simulink model "EncTest"  (R2022b)
settings: Solver=FixedStepDiscrete  StartTime=0.0  StopTime=inf  FixedStep=0.001  RelTol=1e-3
settings Model: DataDictionary=MCU_Input_Sldd.sldd  Creator=ZYH  LastModifiedBy=ZYH
settings OptimizationCC: DefaultParameterBehavior=Inlined  DefaultUnderspecifiedDataType=single  EnhancedBackFolding=on  PassReuseOutputArgsAs=Individual arguments  ZeroExternalMemoryAtStartup=off  ZeroInternalMemoryAtStartup=off  OptimizeBlockOrder=speed  DifferentSizesBufferReuse=on  OptimizationCustomize=off  EfficientTunableParamExpr=on
settings DebuggingCC: ParameterTunabilityLossMsg=error
settings SFSimCC: MATLABDynamicMemAlloc=off
settings RTWCC: Description=Embedded Coder  SystemTargetFile=ert.tlc  GenCodeOnly=on  TemplateMakefile=ert_default_tmf
settings CodeAppCC: IgnoreCustomStorageClasses=off  MaxIdLength=40  OperatorAnnotations=on  SimulinkDataObjDesc=on  SFDataObjDesc=on  SimulinkBlockComments=off
settings ERTTargetCC: TargetLangStandard=C99 (ISO)  GenerateSampleERTMain=on  InlinedParameterPlacement=NonHierarchical  ERTCustomFileTemplate=example_file_process.tlc

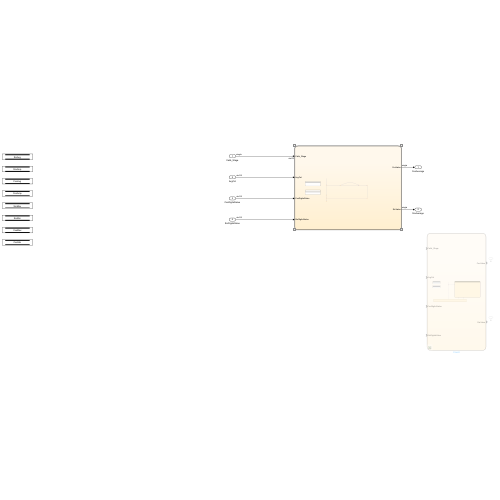
[thumbnail: Simulink's stored preview of the top-level diagram]
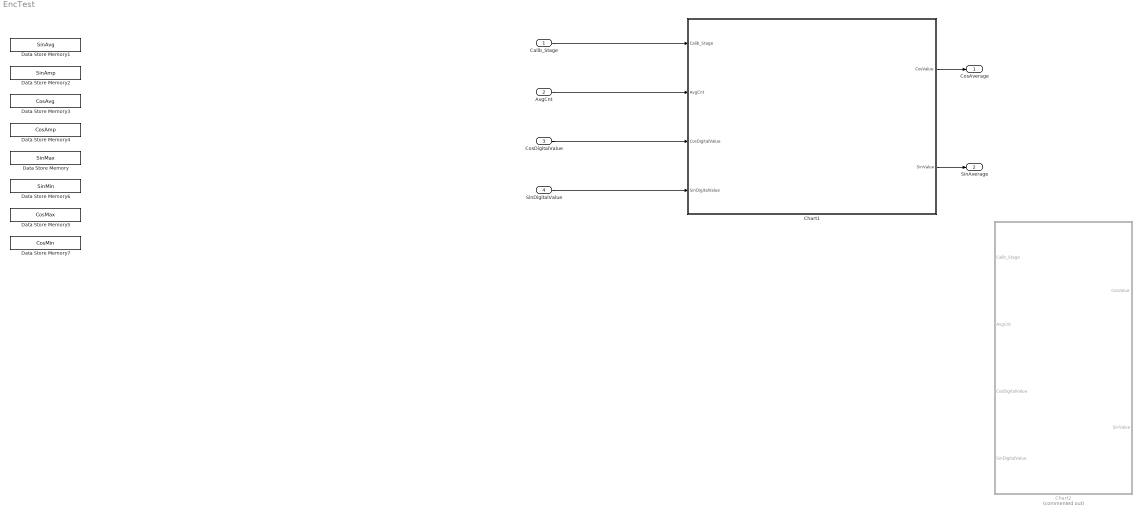
== system EncTest ==
  Calib_Stage : Inport
  AvgCnt : Inport  Port=2
  CosDigitalValue : Inport  Port=3
  SinDigitalValue : Inport  Port=4
  Chart1 : Stateflow chart  TreatAsAtomicUnit=on
      settings: RTWSystemCode=Nonreusable function
  Chart2 : Stateflow chart  Commented=on  TreatAsAtomicUnit=on
      settings: RTWSystemCode=Nonreusable function
  Data Store Memory : DataStoreMemory  DataStoreName=SinMax  WriteAfterWriteMsg=warning  InitialValue=2048  ShowAdditionalParam=off
  Data Store Memory1 : DataStoreMemory  DataStoreName=SinAvg  WriteAfterWriteMsg=warning  InitialValue=ParamCfg_Sinavg_u16  ShowAdditionalParam=off  OutDataTypeStr=uint16  StateMustResolveToSignalObject=on
  Data Store Memory2 : DataStoreMemory  DataStoreName=SinAmp  WriteAfterWriteMsg=warning  InitialValue=ParamCfg_Sinamp_u16  ShowAdditionalParam=off  OutDataTypeStr=uint16  StateMustResolveToSignalObject=on
  Data Store Memory3 : DataStoreMemory  DataStoreName=CosAvg  WriteAfterWriteMsg=warning  InitialValue=ParamCfg_Cosavg_u16  ShowAdditionalParam=off  OutDataTypeStr=uint16  StateMustResolveToSignalObject=on
  Data Store Memory4 : DataStoreMemory  DataStoreName=CosAmp  WriteAfterWriteMsg=warning  InitialValue=ParamCfg_Cosamp_u16  ShowAdditionalParam=off  OutDataTypeStr=uint16  StateMustResolveToSignalObject=on
  Data Store Memory5 : DataStoreMemory  DataStoreName=CosMax  WriteAfterWriteMsg=warning  InitialValue=2048  ShowAdditionalParam=off
  Data Store Memory6 : DataStoreMemory  DataStoreName=SinMin  WriteAfterWriteMsg=warning  InitialValue=2048  ShowAdditionalParam=off
  Data Store Memory7 : DataStoreMemory  DataStoreName=CosMin  WriteAfterWriteMsg=warning  InitialValue=2048  ShowAdditionalParam=off
  CosAverage : Outport
  SinAverage : Outport  Port=2
  wires:
  Chart1/1(CosValue) -> CosAverage/1
  Chart1/2(SinValue) -> SinAverage/1
  Calib_Stage/1 -> Chart1/1(Calib_Stage)
  AvgCnt/1 -> Chart1/2(AvgCnt)
  CosDigitalValue/1 -> Chart1/3(CosDigitalValue)
  SinDigitalValue/1 -> Chart1/4(SinDigitalValue)

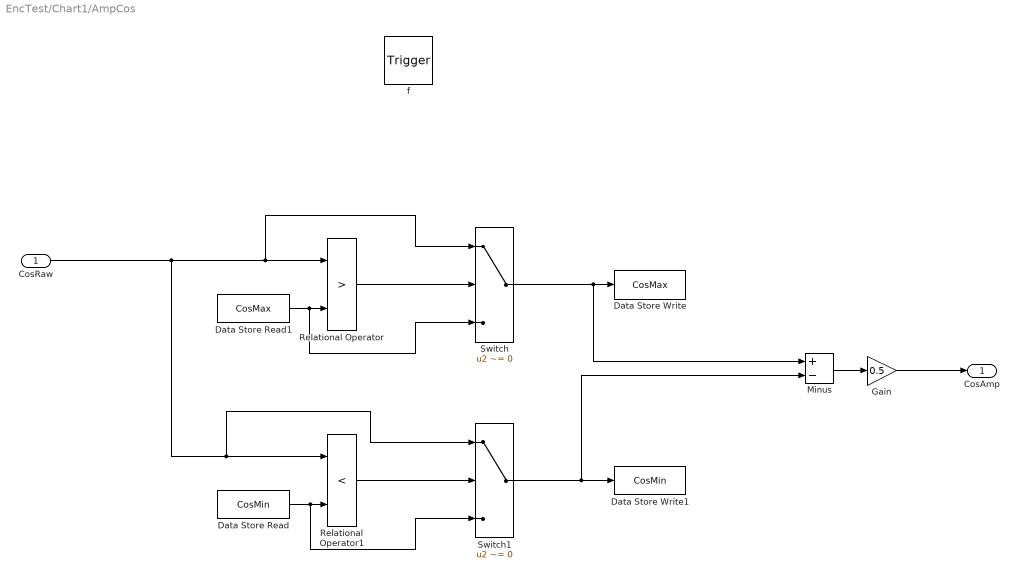
== system EncTest/Chart1/AmpCos ==
  CosRaw : Inport  OutDataTypeStr=uint16  PortDimensions=1
  f : TriggerPort  TriggerType=function-call  VariantControl=(inherit)
      settings: CopyFcn=Stateflow.SLINSF.SimulinkMan.removeBlockPreDeleteFcn  PreDeleteFcn=Stateflow.SLINSF.SimulinkMan.unsafePredeleteFcn
  Data Store Read : DataStoreRead  DataStoreName=CosMin  IndexOptions=Index vector (dialog)  Indices=1  OutputSizes=1
  Data Store Read1 : DataStoreRead  DataStoreName=CosMax  IndexOptions=Index vector (dialog)  Indices=1  OutputSizes=1
  Data Store Write : DataStoreWrite  DataStoreName=CosMax  IndexOptions=Index vector (dialog)  Indices=1  OutputSizes=1
  Data Store Write1 : DataStoreWrite  DataStoreName=CosMin  IndexOptions=Index vector (dialog)  Indices=1  OutputSizes=1
  Gain : Gain  Gain=0.5  ParamDataTypeStr=single  OutDataTypeStr=single
  Minus : Sum  Inputs=+-
  Relational Operator : RelationalOperator  Operator=>  OutDataTypeStr=boolean  RndMeth=Simplest  InputSameDT=off
  Relational Operator1 : RelationalOperator  Operator=<  OutDataTypeStr=boolean  RndMeth=Simplest  InputSameDT=off
  Switch : Switch  Criteria=u2 ~= 0  SaturateOnIntegerOverflow=off  InputSameDT=off
  Switch1 : Switch  Criteria=u2 ~= 0  SaturateOnIntegerOverflow=off  InputSameDT=off
  CosAmp : Outport  OutDataTypeStr=single
  wires:
  CosRaw/1 -> Switch1/1, Relational Operator1/1, Switch/1, Relational Operator/1
  Data Store Read1/1 -> Switch/3, Relational Operator/2
  Relational Operator/1 -> Switch/2
  Switch/1 -> Minus/1, Data Store Write/1
  Data Store Read/1 -> Switch1/3, Relational Operator1/2
  Relational Operator1/1 -> Switch1/2
  Switch1/1 -> Minus/2, Data Store Write1/1
  Minus/1 -> Gain/1
  Gain/1 -> CosAmp/1

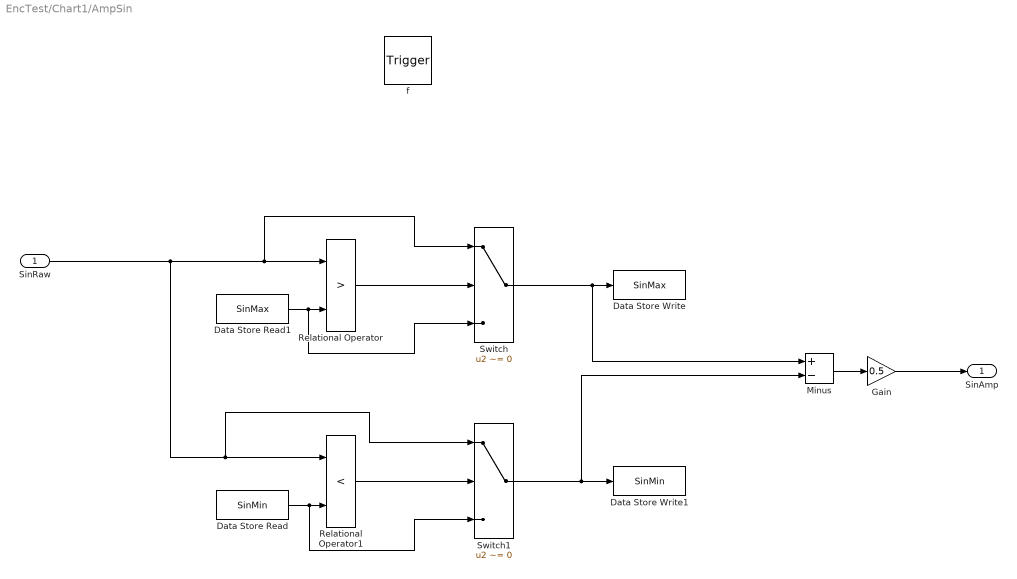
== system EncTest/Chart1/AmpSin ==
  SinRaw : Inport  OutDataTypeStr=uint16  PortDimensions=1
  f : TriggerPort  TriggerType=function-call  VariantControl=(inherit)
      settings: CopyFcn=Stateflow.SLINSF.SimulinkMan.removeBlockPreDeleteFcn  PreDeleteFcn=Stateflow.SLINSF.SimulinkMan.unsafePredeleteFcn
  Data Store Read : DataStoreRead  DataStoreName=SinMin  IndexOptions=Index vector (dialog)  Indices=1  OutputSizes=1
  Data Store Read1 : DataStoreRead  DataStoreName=SinMax  IndexOptions=Index vector (dialog)  Indices=1  OutputSizes=1
  Data Store Write : DataStoreWrite  DataStoreName=SinMax  IndexOptions=Index vector (dialog)  Indices=1  OutputSizes=1
  Data Store Write1 : DataStoreWrite  DataStoreName=SinMin  IndexOptions=Index vector (dialog)  Indices=1  OutputSizes=1
  Gain : Gain  Gain=0.5  ParamDataTypeStr=single  OutDataTypeStr=single
  Minus : Sum  Inputs=+-
  Relational Operator : RelationalOperator  Operator=>  OutDataTypeStr=boolean  RndMeth=Simplest  InputSameDT=off
  Relational Operator1 : RelationalOperator  Operator=<  OutDataTypeStr=boolean  RndMeth=Simplest  InputSameDT=off
  Switch : Switch  Criteria=u2 ~= 0  SaturateOnIntegerOverflow=off  InputSameDT=off
  Switch1 : Switch  Criteria=u2 ~= 0  SaturateOnIntegerOverflow=off  InputSameDT=off
  SinAmp : Outport  OutDataTypeStr=single  PortDimensions=1
  wires:
  SinRaw/1 -> Switch1/1, Relational Operator1/1, Switch/1, Relational Operator/1
  Data Store Read1/1 -> Switch/3, Relational Operator/2
  Relational Operator/1 -> Switch/2
  Switch/1 -> Minus/1, Data Store Write/1
  Data Store Read/1 -> Switch1/3, Relational Operator1/2
  Relational Operator1/1 -> Switch1/2
  Switch1/1 -> Minus/2, Data Store Write1/1
  Minus/1 -> Gain/1
  Gain/1 -> SinAmp/1

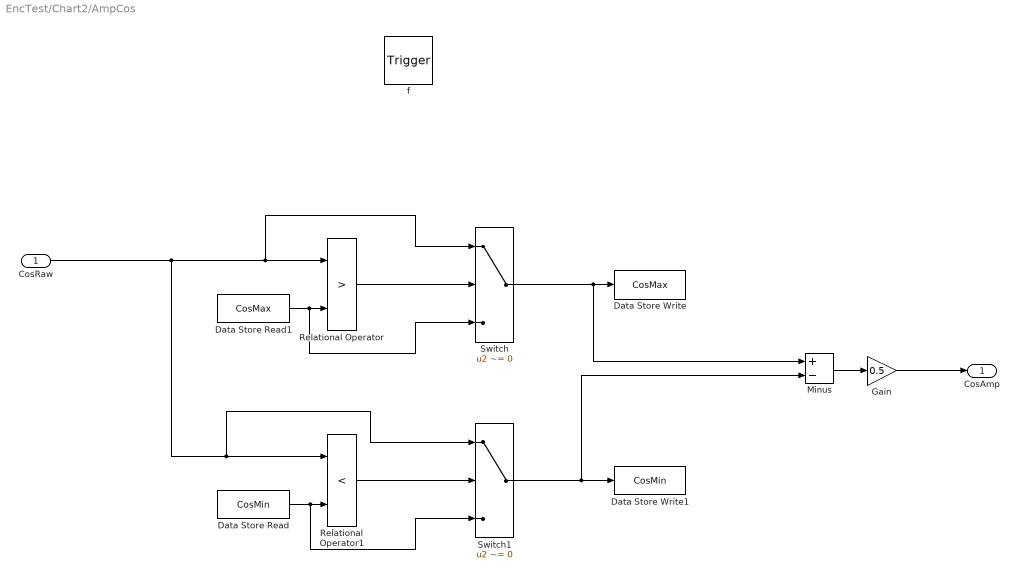
== system EncTest/Chart2/AmpCos ==
  CosRaw : Inport  OutDataTypeStr=uint16  PortDimensions=1
  f : TriggerPort  TriggerType=function-call  VariantControl=(inherit)
      settings: CopyFcn=Stateflow.SLINSF.SimulinkMan.removeBlockPreDeleteFcn  PreDeleteFcn=Stateflow.SLINSF.SimulinkMan.unsafePredeleteFcn
  Data Store Read : DataStoreRead  DataStoreName=CosMin  IndexOptions=Index vector (dialog)  Indices=1  OutputSizes=1
  Data Store Read1 : DataStoreRead  DataStoreName=CosMax  IndexOptions=Index vector (dialog)  Indices=1  OutputSizes=1
  Data Store Write : DataStoreWrite  DataStoreName=CosMax  IndexOptions=Index vector (dialog)  Indices=1  OutputSizes=1
  Data Store Write1 : DataStoreWrite  DataStoreName=CosMin  IndexOptions=Index vector (dialog)  Indices=1  OutputSizes=1
  Gain : Gain  Gain=0.5  ParamDataTypeStr=single  OutDataTypeStr=single
  Minus : Sum  Inputs=+-
  Relational Operator : RelationalOperator  Operator=>  OutDataTypeStr=boolean  RndMeth=Simplest  InputSameDT=off
  Relational Operator1 : RelationalOperator  Operator=<  OutDataTypeStr=boolean  RndMeth=Simplest  InputSameDT=off
  Switch : Switch  Criteria=u2 ~= 0  SaturateOnIntegerOverflow=off  InputSameDT=off
  Switch1 : Switch  Criteria=u2 ~= 0  SaturateOnIntegerOverflow=off  InputSameDT=off
  CosAmp : Outport  OutDataTypeStr=single
  wires:
  CosRaw/1 -> Switch1/1, Relational Operator1/1, Switch/1, Relational Operator/1
  Data Store Read1/1 -> Switch/3, Relational Operator/2
  Relational Operator/1 -> Switch/2
  Switch/1 -> Minus/1, Data Store Write/1
  Data Store Read/1 -> Switch1/3, Relational Operator1/2
  Relational Operator1/1 -> Switch1/2
  Switch1/1 -> Minus/2, Data Store Write1/1
  Minus/1 -> Gain/1
  Gain/1 -> CosAmp/1

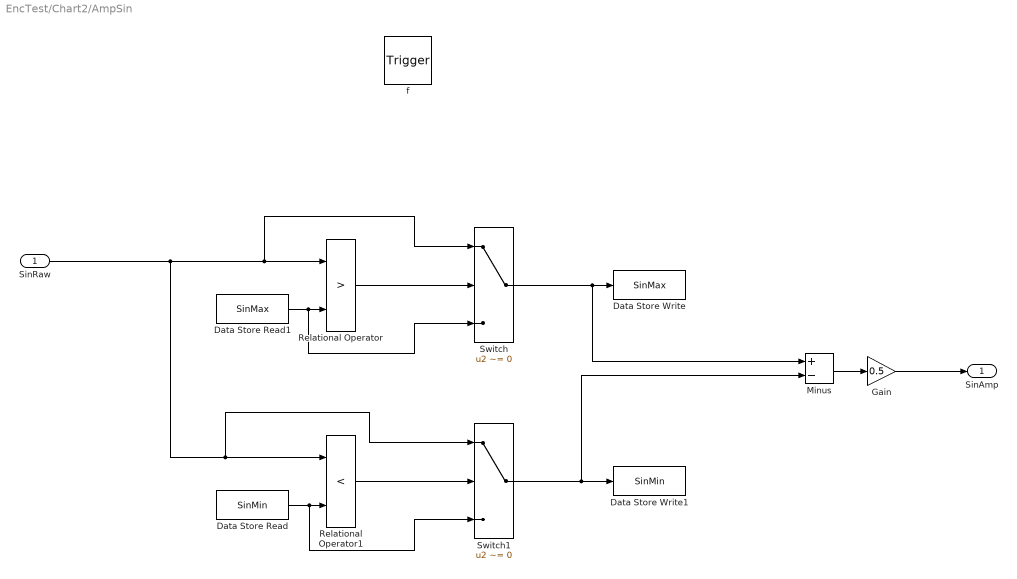
== system EncTest/Chart2/AmpSin ==
  SinRaw : Inport  OutDataTypeStr=uint16  PortDimensions=1
  f : TriggerPort  TriggerType=function-call  VariantControl=(inherit)
      settings: CopyFcn=Stateflow.SLINSF.SimulinkMan.removeBlockPreDeleteFcn  PreDeleteFcn=Stateflow.SLINSF.SimulinkMan.unsafePredeleteFcn
  Data Store Read : DataStoreRead  DataStoreName=SinMin  IndexOptions=Index vector (dialog)  Indices=1  OutputSizes=1
  Data Store Read1 : DataStoreRead  DataStoreName=SinMax  IndexOptions=Index vector (dialog)  Indices=1  OutputSizes=1
  Data Store Write : DataStoreWrite  DataStoreName=SinMax  IndexOptions=Index vector (dialog)  Indices=1  OutputSizes=1
  Data Store Write1 : DataStoreWrite  DataStoreName=SinMin  IndexOptions=Index vector (dialog)  Indices=1  OutputSizes=1
  Gain : Gain  Gain=0.5  ParamDataTypeStr=single  OutDataTypeStr=single
  Minus : Sum  Inputs=+-
  Relational Operator : RelationalOperator  Operator=>  OutDataTypeStr=boolean  RndMeth=Simplest  InputSameDT=off
  Relational Operator1 : RelationalOperator  Operator=<  OutDataTypeStr=boolean  RndMeth=Simplest  InputSameDT=off
  Switch : Switch  Criteria=u2 ~= 0  SaturateOnIntegerOverflow=off  InputSameDT=off
  Switch1 : Switch  Criteria=u2 ~= 0  SaturateOnIntegerOverflow=off  InputSameDT=off
  SinAmp : Outport  OutDataTypeStr=single  PortDimensions=1
  wires:
  SinRaw/1 -> Switch1/1, Relational Operator1/1, Switch/1, Relational Operator/1
  Data Store Read1/1 -> Switch/3, Relational Operator/2
  Relational Operator/1 -> Switch/2
  Switch/1 -> Minus/1, Data Store Write/1
  Data Store Read/1 -> Switch1/3, Relational Operator1/2
  Relational Operator1/1 -> Switch1/2
  Switch1/1 -> Minus/2, Data Store Write1/1
  Minus/1 -> Gain/1
  Gain/1 -> SinAmp/1

== stateflow chart EncTest/Chart1 ==
  state SinAmp = AmpSin(SinRaw) [function]
  state CosAmp = AmpCos(CosRaw) [function]
  (default) -> (junction 94)
  (junction 108) -> (junction 99) [order 1] : [Cnt < AvgCnt]{
      | SinAmplitude =AmpSin(SinDigitalValue);
      | CosAmplitude = AmpCos(CosDigitalValue);
      | SinSum = SinSum + SinDigitalValue;
      | CosSum = CosSum + CosDigitalValue;
      | Cnt = Cnt+1;
      | }
  (junction 94) -> (junction 108) [order 1] : [Calib_Stage == NORMALIZE]
  (junction 108) -> (junction 99) [order 2]
  (junction 99) -> (junction 117)
  (junction 94) -> (junction 100) [order 2] : {SinSum = 0;
      | CosSum= 0;
      | Cnt = 0;
      | ToFinish = 0;
      | SinValue = (SinDigitalValue-SinAverage)*SinAmplitudeInverse;
      | CosValue = (CosDigitalValue - CosAverage)*CosAmplitudeInverse;
      | }
  (junction 117) -> (junction 95) : {
      |     %求均值
      |     SinAverage = SinSum/(Cnt);
      |     CosAverage = CosSum/(Cnt);
      |
      |     %求幅值倒数
      |     SinAmplitudeInverse = 1/SinAmplitude;
      |     CosAmplitudeInverse = 1/CosAmplitude;
      |
      | %更新参数
      | SinAvg = SinAverage*10;
      | CosAvg = CosAverage *10;
      | SinAmp = SinAmplitude *10;
      | CosAmp = CosAmplitude *10;
      |
      | SinValue = (SinDigitalValue-SinAverage)*SinAmplitudeInverse;
      | CosValue = (CosDigitalValue - CosAverage)*CosAmplitudeInverse;
      | }
  (junction 100) -> (junction 112)
  (junction 95) -> (junction 112) : {SinSum = 0;
      | CosSum= 0;
      | Cnt = 0;
      | ToFinish = 0}
  (junction 112) -> (junction 107)
  data: SinRaw function_input uint16 size=1; SinAmp function_output single size=1; CosRaw function_input uint16 size=1; CosAmp function_output single; Calib_Stage input uint16; AvgCnt input uint16; CosDigitalValue input uint16; SinDigitalValue input uint16; CosValue output single; SinValue output single; Cnt local uint16 =0; CosSum local single; SinSum local single; COMPENSATE constant uint16 =2; NORMALIZE constant uint16 =1; SinAverage local single; CosAverage local single; CosAmplitudeInverse local single; SinAmplitudeInverse local single; CosAmplitude local single; SinAmplitude local single; CosAvg data_store_memory; SinAvg data_store_memory; SinAmp data_store_memory; CosAmp data_store_memory; ToFinish local uint8 =0

== stateflow chart EncTest/Chart2 ==
  state Normalize
    state A
      SinAmplitude =AmpSin(SinDigitalValue);
      CosAmplitude = AmpCos(CosDigitalValue);
      SinSum = SinSum + SinDigitalValue;
      CosSum = CosSum + CosDigitalValue;
      Cnt = Cnt+1;
    state B
      %求均值
      SinAverage = SinSum/(Cnt);
      CosAverage = CosSum/(Cnt);
      %求幅值倒数
      SinAmplitudeInverse = 1/SinAmplitude;
      CosAmplitudeInverse = 1/CosAmplitude;
      %更新参数
      SinAvg = SinAverage*10;
      CosAvg = CosAverage *10;
      SinAmp = SinAmplitude *10;
      CosAmp = CosAmplitude *10;
      %状态跳转
      ToFinish = 1
    (default) -> A
    A -> B : [Cnt > AvgCnt]
  state SinAmp = AmpSin(SinRaw) [function]
  state CosAmp = AmpCos(CosRaw) [function]
  state Finish
    SinSum = 0;
    CosSum= 0;
    Cnt = 0;
    ToFinish = 0;
  (default) -> (junction 7)
  (junction 7) -> Normalize [order 1] : [Calib_Stage == NORMALIZE]
  (junction 7) -> Finish [order 2]
  Normalize -> Finish : [ToFinish == 1]
  Finish -> Normalize : [Calib_Stage == NORMALIZE]
  data: SinRaw function_input uint16 size=1; SinAmp function_output single size=1; CosRaw function_input uint16 size=1; CosAmp function_output single; Calib_Stage input uint16; AvgCnt input uint16; CosDigitalValue input uint16; SinDigitalValue input uint16; CosValue output single; SinValue output single; Cnt local uint16 =0; CosSum local single; SinSum local single; COMPENSATE constant uint16 =2; NORMALIZE constant uint16 =1; SinAverage local single; CosAverage local single; CosAmplitudeInverse local single; SinAmplitudeInverse local single; CosAmplitude local single; SinAmplitude local single; CosAvg data_store_memory; SinAvg data_store_memory; SinAmp data_store_memory; CosAmp data_store_memory; ToFinish local uint8 =0
